simulink model "cnt2019a_new"  (R2019a)
settings: Solver=VariableStepAuto  StartTime=0.0  StopTime=50.0  RelTol=1e-3
settings Model: Creator=Akhil Jarodia  LastModifiedBy=Akhil Jarodia
settings DebuggingCC: UnderSpecifiedDimensionMsg=warning

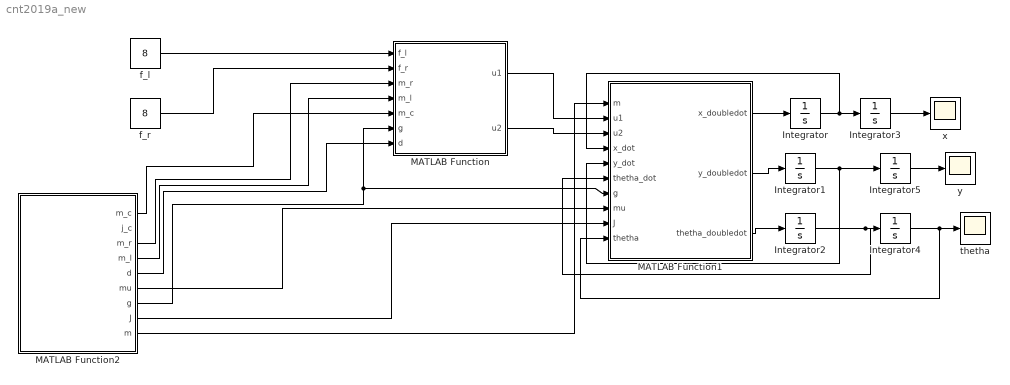
== system cnt2019a_new ==
  Integrator{,1..5} (6 alike) : Integrator
  MATLAB Function : MATLAB Function  TreatAsAtomicUnit=on
  MATLAB Function1 : MATLAB Function  TreatAsAtomicUnit=on
  MATLAB Function2 : MATLAB Function  TreatAsAtomicUnit=on
  f_l : Constant  Value=8
  "f_r " : Constant  Value=8
  thetha : Scope
  x : Scope
  y : Scope
  wires:
  MATLAB Function2/7(g) -> MATLAB Function/6(g), MATLAB Function1/7(g)
  MATLAB Function2/5(d) -> MATLAB Function/7(d)
  MATLAB Function2/8(J) -> MATLAB Function1/9(J)
  f_l/1 -> MATLAB Function/1(f_l)
  "f_r "/1 -> MATLAB Function/2(f_r)
  MATLAB Function2/1(m_c) -> MATLAB Function/5(m_c)
  MATLAB Function2/3(m_r) -> MATLAB Function/3(m_r)
  MATLAB Function2/4(m_l) -> MATLAB Function/4(m_l)
  MATLAB Function/1(u1) -> MATLAB Function1/2(u1)
  MATLAB Function/2(u2) -> MATLAB Function1/3(u2)
  MATLAB Function2/6(mu) -> MATLAB Function1/8(mu)
  MATLAB Function1/2(y_doubledot) -> Integrator1/1
  MATLAB Function1/1(x_doubledot) -> Integrator/1
  MATLAB Function1/3(thetha_doubledot) -> Integrator2/1
  Integrator/1 -> MATLAB Function1/4(x_dot), Integrator3/1
  Integrator1/1 -> Integrator5/1, MATLAB Function1/5(y_dot)
  Integrator2/1 -> MATLAB Function1/6(thetha_dot), Integrator4/1
  Integrator3/1 -> x/1
  Integrator4/1 -> MATLAB Function1/10(thetha), thetha/1
  Integrator5/1 -> y/1
  MATLAB Function2/9(m) -> MATLAB Function1/1(m)

== matlab function cnt2019a_new/MATLAB Function1 ==
  data: m input; u1 input; x_doubledot output; u2 input; x_dot input; y_dot input; thetha_dot input; g input; mu input; y_doubledot output; thetha_doubledot output; J input; thetha input
function [x_doubledot,y_doubledot,thetha_doubledot]= fcn(m,u1,u2,x_dot,y_dot,thetha_dot,g,mu,J,thetha)
temp=[g -1*mu 0 0; 0 0 0 0;0 0 0 0]*[thetha;x_dot ;y_dot ;thetha_dot] + [0 0;1/m 0;0 1/J]*[u1;u2];
% disp(temp);
x_doubledot=temp(1);
y_doubledot=temp(2);
thetha_doubledot=temp(3);

== matlab function cnt2019a_new/MATLAB Function ==
  data: f_l input; u1 output; f_r input; m_r input; m_l input; m_c input; g input; d input; u2 output
function [u1,u2]= fcn(f_l,f_r,m_r,m_l,m_c,g,d)

u1=f_l+f_r-(m_c+m_r+m_l)*g;
u2=(f_l-f_r)*d;

== matlab function cnt2019a_new/MATLAB Function2 ==
  data: m_c output; j_c output; m_r output; m_l output; d output; mu output; g output; J output; m output
function [m_c,j_c,m_r,m_l,d,mu,g,J,m]= constraints
 m_c=1;
 j_c=0.0042;
 m_r=0.25;
 m_l=0.25;
 d=0.3;
 mu=0.1;
 g=9.81;
 J=j_c+2*m_c*d^2;
 m=m_c+m_r+m_l;
